simulink model "DC_Motor_Control_Manual"  (R2025b)
settings: Solver=FixedStepAuto  StartTime=0.0  StopTime=inf  FixedStep=0.02  RelTol=1e-3  EnableMultiTasking=on
libraries: simulink x6, raspberrypiBasiclib x4, raspberrypiNetworklib x1
settings Model: ExtModeTrigDuration=2  Creator=jujma  LastModifiedBy=jujma
settings SolverCC: PositivePriorityOrder=on
settings OptimizationCC: EnhancedBackFolding=on  PassReuseOutputArgsAs=Individual arguments  ZeroExternalMemoryAtStartup=off  ZeroInternalMemoryAtStartup=off  MaxStackSize=200000  OptimizeBlockOrder=speed  DifferentSizesBufferReuse=on  OptimizationCustomize=off  EfficientTunableParamExpr=on
settings DebuggingCC: ParameterTunabilityLossMsg=error
settings HardwareCC: ProdBitPerPointer=32.0  ProdBitPerSizeT=32.0  ProdBitPerPtrDiffT=32.0  ProdLargestAtomicInteger=Long  ProdLargestAtomicFloat=Double  ProdWordSize=32.0  ProdLongLongMode=on  ProdHWDeviceType=ARM Compatible->ARM Cortex-A (32-bit)
settings RTWCC: SystemTargetFile=ert.tlc  HardwareBoard=Raspberry Pi  TLCOptions="-aInlineSetEventsForThisBaseRateFcn=TLC_FALSE -aSuppressMultiTaskScheduler=TLC_FALSE  -aRateBasedStepFcn=0"  TemplateMakefile=ert_default_tmf  Toolchain=GNU GCC Embedded Linux  BuildConfiguration=Faster Runs  Description=Embedded Coder
settings CodeAppCC: ForceParamTrailComments=on  IgnoreCustomStorageClasses=off  OperatorAnnotations=on  SimulinkDataObjDesc=on  SFDataObjDesc=on  InsertBlockDesc=on
settings ERTTargetCC: ExtModeTransport=2.0  ExtModeStaticAlloc=on  ExtModeMexFile=ext_xcp  ExtModeIntrfLevel=Level2 - Open  InlinedParameterPlacement=Hierarchical  CodeReplacementLibrary=ARM Cortex-A CMSIS  SupportVariableSizeSignals=on

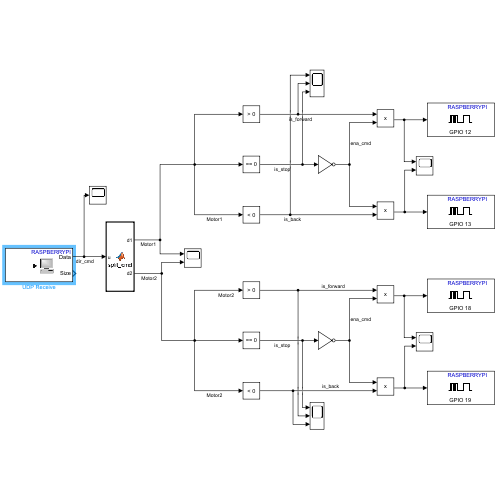
[thumbnail: Simulink's stored preview of the top-level diagram]
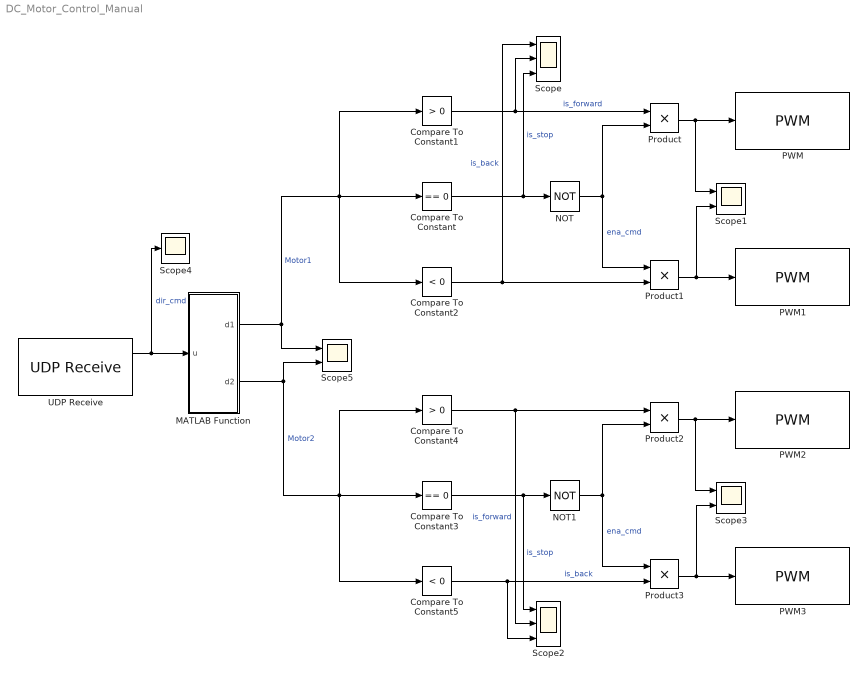
== system DC_Motor_Control_Manual ==
  Compare To Constant : simulink/Logic and Bit Operations/Compare To Constant  relop===  const=0  OutDataTypeStr=boolean
  Compare To Constant1 : simulink/Logic and Bit Operations/Compare To Constant  relop=>  const=0  OutDataTypeStr=boolean
  Compare To Constant2 : simulink/Logic and Bit Operations/Compare To Constant  relop=<  const=0  OutDataTypeStr=boolean
  Compare To Constant3 : simulink/Logic and Bit Operations/Compare To Constant  relop===  const=0  OutDataTypeStr=boolean
  Compare To Constant4 : simulink/Logic and Bit Operations/Compare To Constant  relop=>  const=0  OutDataTypeStr=boolean
  Compare To Constant5 : simulink/Logic and Bit Operations/Compare To Constant  relop=<  const=0  OutDataTypeStr=boolean
  MATLAB Function : MATLAB Function  TreatAsAtomicUnit=on
  NOT : Logic  Operator=NOT  IconShape=distinctive  AllPortsSameDT=off  OutDataTypeStr=boolean
  NOT1 : Logic  Operator=NOT  IconShape=distinctive  AllPortsSameDT=off  OutDataTypeStr=boolean
  PWM : raspberrypiBasiclib/PWM  board=Pi Zero W  Pin_=12  Frequency=500  blockPlatform=Raspberry Pi
  PWM1 : raspberrypiBasiclib/PWM  board=Pi Zero W  Pin_=13  Frequency=500  blockPlatform=Raspberry Pi
  PWM2 : raspberrypiBasiclib/PWM  board=Pi Zero W  Pin_=18  Frequency=500  blockPlatform=Raspberry Pi
  PWM3 : raspberrypiBasiclib/PWM  board=Pi Zero W  Pin_=19  Frequency=500  blockPlatform=Raspberry Pi
  Product{,1..3} (4 alike) : Product
  Scope : Scope  NumInputPorts=3
      settings: ActiveDisplayYMinimum=-0.12499999999999997  ActiveDisplayYMaximum=1.125
  Scope1 : Scope  NumInputPorts=2
      settings: ActiveDisplayYMinimum=-16.578406132891736  ActiveDisplayYMaximum=15.421593867108266
  Scope2 : Scope  NumInputPorts=3
      settings: ActiveDisplayYMinimum=-0.12499999999999997  ActiveDisplayYMaximum=1.125  DataLoggingVariableName=ScopeData2
  Scope3 : Scope  NumInputPorts=2
      settings: ActiveDisplayYMinimum=-16.578406132891736  ActiveDisplayYMaximum=15.421593867108266  DataLoggingVariableName=ScopeData3
  Scope4 : Scope
      settings: ActiveDisplayYMinimum=-1.25  ActiveDisplayYMaximum=1.25  DataLoggingVariableName=ScopeData4
  Scope5 : Scope  NumInputPorts=2
      settings: ActiveDisplayYMinimum=-1.25  ActiveDisplayYMaximum=1.25  DataLoggingVariableName=ScopeData5
  UDP Receive : raspberrypiNetworklib/UDP Receive  localURL='0.0.0.0'  localPort=55001  remoteURL='0.0.0.0'  remotePort=-1  recvBufferSize=8192  signalDatatype=double  dims=2  isVarSize=off  showBlockingTime=off  blockingTime=0  sampletime=0.02  blockPlatform=Raspberry Pi
  wires:
  NOT/1 -> Product/2, Product1/1  "ena_cmd"
  Compare To Constant/1 -> Scope/3, NOT/1  "is_stop"
  Compare To Constant1/1 -> Scope/2, Product/1  "is_forward"
  MATLAB Function/1(d1) -> Scope5/1, Compare To Constant1/1, Compare To Constant2/1, Compare To Constant/1  "Motor1"
  Compare To Constant2/1 -> Scope/1, Product1/2  "is_back"
  Product1/1 -> Scope1/2, PWM1/1
  Product/1 -> Scope1/1, PWM/1
  UDP Receive/1 -> MATLAB Function/1(u), Scope4/1  "dir_cmd"
  Compare To Constant4/1 -> Scope2/2, Product2/1  "is_forward"
  NOT1/1 -> Product2/2, Product3/1  "ena_cmd"
  Product3/1 -> Scope3/2, PWM3/1
  Product2/1 -> Scope3/1, PWM2/1
  Compare To Constant5/1 -> Scope2/3, Product3/2  "is_back"
  Compare To Constant3/1 -> Scope2/1, NOT1/1  "is_stop"
  MATLAB Function/2(d2) -> Compare To Constant4/1, Compare To Constant5/1, Compare To Constant3/1, Scope5/2  "Motor2"

== matlab function DC_Motor_Control_Manual/MATLAB Function ==
  data: u input; d1 output; d2 output
function [d1, d2] = split_cmd(u)
%#codegen
% u is a 1x2 vector: [dir1 dir2]
d1 = u(1);
d2 = u(2);
end
